simulink model "siasun_config_casadi_VS_lsj_sim_16a"  (R2020a)
settings: Solver=FixedStepAuto  StartTime=0.0  StopTime=20  FixedStep=0.001  RelTol=1e-3  EnableMultiTasking=on
values from neighbouring files (symbols this model uses):
  a1 = 0.040    (= 0.04)    [set_mode_parameter_siasun.m]
  a2 = 0.275    [set_mode_parameter_siasun.m]
  a3 = 0.025    [set_mode_parameter_siasun.m]
  d1 = 0.342    [set_mode_parameter_siasun.m]
  d4 = 0.280    (= 0.28)    [set_mode_parameter_siasun.m]
  fc1 = 0    [set_mode_parameter_siasun.m]
  fc2 = 0    [set_mode_parameter_siasun.m]
  fc3 = 0    [set_mode_parameter_siasun.m]
  fc4 = 0    [set_mode_parameter_siasun.m]
  fc5 = 0    [set_mode_parameter_siasun.m]
  fc6 = 0    [set_mode_parameter_siasun.m]
  fv1 = 0    [set_mode_parameter_siasun.m]
  fv2 = 0    [set_mode_parameter_siasun.m]
  fv3 = 0    [set_mode_parameter_siasun.m]
  fv4 = 0    [set_mode_parameter_siasun.m]
  fv5 = 0    [set_mode_parameter_siasun.m]
  fv6 = 0    [set_mode_parameter_siasun.m]
  Ia1 = 0    [set_mode_parameter_siasun.m]
  Ia2 = 0    [set_mode_parameter_siasun.m]
  Ia3 = 0    [set_mode_parameter_siasun.m]
  Ia4 = 0    [set_mode_parameter_siasun.m]
  Ia5 = 0    [set_mode_parameter_siasun.m]
  Ia6 = 0    [set_mode_parameter_siasun.m]
  Ic111 = 0    [set_mode_parameter_siasun.m]
  Ic112 = 0    [set_mode_parameter_siasun.m]
  Ic113 = 0    [set_mode_parameter_siasun.m]
  Ic122 = 0    [set_mode_parameter_siasun.m]
  Ic123 = 0    [set_mode_parameter_siasun.m]
  Ic133 = 1.3676    [set_mode_parameter_siasun.m]
  Ic211 = 8.8194    [set_mode_parameter_siasun.m]
  Ic212 = 0    [set_mode_parameter_siasun.m]
  Ic213 = 0    [set_mode_parameter_siasun.m]
  Ic222 = 6.0549    [set_mode_parameter_siasun.m]
  Ic223 = 0    [set_mode_parameter_siasun.m]
  Ic233 = 0.9569    [set_mode_parameter_siasun.m]
  Ic311 = 0.0332    [set_mode_parameter_siasun.m]
  Ic312 = 0    [set_mode_parameter_siasun.m]
  Ic313 = 0    [set_mode_parameter_siasun.m]
  Ic322 = 1.8442    [set_mode_parameter_siasun.m]
  Ic323 = 0    [set_mode_parameter_siasun.m]
  Ic333 = 1.0560    (= 1.056)    [set_mode_parameter_siasun.m]
  Ic411 = 0.1448    [set_mode_parameter_siasun.m]
  Ic412 = 0    [set_mode_parameter_siasun.m]
  Ic413 = 0    [set_mode_parameter_siasun.m]
  Ic422 = 0.0015    [set_mode_parameter_siasun.m]
  Ic423 = 0    [set_mode_parameter_siasun.m]
  Ic433 = 0.0822    [set_mode_parameter_siasun.m]
  Ic511 = 0    [set_mode_parameter_siasun.m]
  Ic512 = 0    [set_mode_parameter_siasun.m]
  Ic513 = 0    [set_mode_parameter_siasun.m]
  Ic522 = 0.0121    [set_mode_parameter_siasun.m]
  Ic523 = 0    [set_mode_parameter_siasun.m]
  Ic533 = 0.0299    [set_mode_parameter_siasun.m]
  Ic611 = 0.0134    [set_mode_parameter_siasun.m]
  Ic612 = 0    [set_mode_parameter_siasun.m]
  Ic613 = 0    [set_mode_parameter_siasun.m]
  Ic622 = 0    [set_mode_parameter_siasun.m]
  Ic623 = 0    [set_mode_parameter_siasun.m]
  Ic633 = 0.0051    [set_mode_parameter_siasun.m]
  m1 = 0.167    [set_mode_parameter_siasun.m]
  m2 = 1    [set_mode_parameter_siasun.m]
  m3 = 0.5    [set_mode_parameter_siasun.m]
  m4 = 0.333    [set_mode_parameter_siasun.m]
  m5 = 0.25    [set_mode_parameter_siasun.m]
  m6 = 0.2    [set_mode_parameter_siasun.m]
  mc11 = 0    [set_mode_parameter_siasun.m]
  mc12 = 0    [set_mode_parameter_siasun.m]
  mc13 = 0.2    [set_mode_parameter_siasun.m]
  mc21 = 0.1291    [set_mode_parameter_siasun.m]
  mc22 = 0    [set_mode_parameter_siasun.m]
  mc23 = 3.3117    [set_mode_parameter_siasun.m]
  mc31 = 1.6484    [set_mode_parameter_siasun.m]
  mc32 = 0    [set_mode_parameter_siasun.m]
  mc33 = 0.8748    [set_mode_parameter_siasun.m]
  mc41 = 0.3200    (= 0.32)    [set_mode_parameter_siasun.m]
  mc42 = 0.2324    [set_mode_parameter_siasun.m]
  mc43 = 0.7083    [set_mode_parameter_siasun.m]
  mc51 = 0.4574    [set_mode_parameter_siasun.m]
  mc52 = 0    [set_mode_parameter_siasun.m]
  mc53 = 0.6427    [set_mode_parameter_siasun.m]
  mc61 = 0.3200    (= 0.32)    [set_mode_parameter_siasun.m]
  mc62 = -0.0513    [set_mode_parameter_siasun.m]
  mc63 = 0.6417    [set_mode_parameter_siasun.m]
undefined symbols (not defined in the file or in its folder): X, Y, Z
libraries: sm_lib x224, nesl_utility x124, simulink x8
(part 6 of 11)

== system siasun_config_casadi_VS_lsj_sim_16a/xb4_rel/Robot/Robot/robot/link6 ==
  Inertia : sm_lib/Body Elements/Inertia  InertiaType=Custom  Mass=m6  MassUnits=kg  CenterOfMass=[mc61 mc62 mc63]  CenterOfMassUnits=m  MomentsOfInertia=[Ic611 Ic622 Ic633 ]  MomentsOfInertiaUnits=kg*m^2  ProductsOfInertia=[Ic623 Ic613 Ic612]  ProductsOfInertiaUnits=kg*m^2  GraphicType=Marker  MarkerShape=Inertia  MarkerSize=20  GraphicVisPropType=SimpleVisualProperties  GraphicDiffuseColor=[0.5 0.5 0.5]  GraphicSpecularColor=[0.5 0.5 0.5 1.0]  GraphicAmbientColor=[0.15 0.15 0.15 1.0]  GraphicEmissiveColor=[0.0 0.0 0.0 1.0]  GraphicShininess=75  GraphicOpacity=1.0
  Reference Frame : sm_lib/Frames and Transforms/Reference Frame
  base : sm_lib/Body Elements/File Solid  ExtGeomFileName=XB4_Model\XB4-6.STL  UnitType=Custom  ExtGeomFileUnits=mm  StepReaderType=HEX  ExportConvexHullGeometry=off  InertiaType=Custom  Mass=0  MassUnits=kg  CenterOfMass=[0 0 0]  CenterOfMassUnits=m  MomentsOfInertia=[0 0 0]  MomentsOfInertiaUnits=kg*m^2  ProductsOfInertia=[0 0 0]  ProductsOfInertiaUnits=kg*m^2  BasedOnType=Density  Density=1000  DensityUnits=kg/(m^3)  DoExposeReferenceFrame=on  SerializedFrames=<Frames/>  GraphicType=FromGeometry  MarkerShape=Sphere  MarkerSize=10  GraphicVisPropType=SimpleVisualProperties  GraphicDiffuseColor=[0.5 0.5 0.5]  GraphicSpecularColor=[0.5 0.5 0.5 1.0]  GraphicAmbientColor=[0.15 0.15 0.15 1.0]  GraphicEmissiveColor=[0.0 0.0 0.0 1.0]  GraphicShininess=75  GraphicOpacity=1.0
  joint1_OriginTransform1 : sm_lib/Frames and Transforms/Rigid Transform  TranslationMethod=Cartesian  TranslationStandardOffset=0  TranslationLengthUnit=m  TranslationStandardAxis=+Z  TranslationCartesianOffset=[0 0 d1]  TranslationROffset=0  TranslationROffsetUnits=m  TranslationZOffset=0  TranslationZOffsetUnits=m  TranslationThetaOffset=0  TranslationThetaOffsetUnits=deg  RotationMethod=RotationSequence  RotationAngleUnits=deg  RotationStandardAxis=+Z  RotationAngle=0.0  RotationArbitraryAxis=[0 0 1]  FollAlignAxisA=+X  BaseAlignAxisA=+Y  FollAlignAxisB=+Y  BaseAlignAxisB=+Z  RotationSequenceAxes=BaseAxes  RotationSequence=XYZ  RotationSequenceAngles=[0 0 0]  RotationSequenceAnglesUnits=rad  RotationMatrix=[1 0 0; 0 1 0; 0 0 1]
  joint2_OriginTransform1 : sm_lib/Frames and Transforms/Rigid Transform  TranslationMethod=Cartesian  TranslationStandardOffset=0  TranslationLengthUnit=m  TranslationStandardAxis=+Z  TranslationCartesianOffset=[a1 0 0]  TranslationROffset=0  TranslationROffsetUnits=m  TranslationZOffset=0  TranslationZOffsetUnits=m  TranslationThetaOffset=0  TranslationThetaOffsetUnits=deg  RotationMethod=RotationSequence  RotationAngleUnits=deg  RotationStandardAxis=+Z  RotationAngle=0.0  RotationArbitraryAxis=[0 0 1]  FollAlignAxisA=+X  BaseAlignAxisA=+Y  FollAlignAxisB=+Y  BaseAlignAxisB=+Z  RotationSequenceAxes=FollowerAxes  RotationSequence=XYZ  RotationSequenceAngles=[-pi/2 0 -pi/2]  RotationSequenceAnglesUnits=rad  RotationMatrix=[1 0 0; 0 1 0; 0 0 1]
  joint3_OriginTransform1 : sm_lib/Frames and Transforms/Rigid Transform  TranslationMethod=Cartesian  TranslationStandardOffset=0  TranslationLengthUnit=m  TranslationStandardAxis=+Z  TranslationCartesianOffset=[a2 0 0]  TranslationROffset=0  TranslationROffsetUnits=m  TranslationZOffset=0  TranslationZOffsetUnits=m  TranslationThetaOffset=0  TranslationThetaOffsetUnits=deg  RotationMethod=RotationSequence  RotationAngleUnits=deg  RotationStandardAxis=+Z  RotationAngle=0.0  RotationArbitraryAxis=[0 0 1]  FollAlignAxisA=+X  BaseAlignAxisA=+Y  FollAlignAxisB=+Y  BaseAlignAxisB=+Z  RotationSequenceAxes=FollowerAxes  RotationSequence=XYZ  RotationSequenceAngles=[0 0 0]  RotationSequenceAnglesUnits=rad  RotationMatrix=[1 0 0; 0 1 0; 0 0 1]
  joint4_AxisInvTransform : sm_lib/Frames and Transforms/Rigid Transform  TranslationMethod=Cartesian  TranslationStandardOffset=0  TranslationLengthUnit=m  TranslationStandardAxis=+Z  TranslationCartesianOffset=[0 0 0]  TranslationROffset=0  TranslationROffsetUnits=m  TranslationZOffset=0  TranslationZOffsetUnits=m  TranslationThetaOffset=0  TranslationThetaOffsetUnits=deg  RotationMethod=RotationSequence  RotationAngleUnits=rad  RotationStandardAxis=+Z  RotationAngle=1.570796  RotationArbitraryAxis=[0 1 0]  FollAlignAxisA=+X  BaseAlignAxisA=+Y  FollAlignAxisB=+Y  BaseAlignAxisB=+Z  RotationSequenceAxes=FollowerAxes  RotationSequence=XYZ  RotationSequenceAngles=[pi/2 0 0]  RotationSequenceAnglesUnits=rad  RotationMatrix=[1 0 0; 0 1 0; 0 0 1]
  joint4_OriginTransform1 : sm_lib/Frames and Transforms/Rigid Transform  TranslationMethod=Cartesian  TranslationStandardOffset=0  TranslationLengthUnit=m  TranslationStandardAxis=+Z  TranslationCartesianOffset=[a3 d4 0]  TranslationROffset=0  TranslationROffsetUnits=m  TranslationZOffset=0  TranslationZOffsetUnits=m  TranslationThetaOffset=0  TranslationThetaOffsetUnits=deg  RotationMethod=RotationSequence  RotationAngleUnits=deg  RotationStandardAxis=+Z  RotationAngle=0.0  RotationArbitraryAxis=[0 0 1]  FollAlignAxisA=+X  BaseAlignAxisA=+Y  FollAlignAxisB=+Y  BaseAlignAxisB=+Z  RotationSequenceAxes=FollowerAxes  RotationSequence=XYZ  RotationSequenceAngles=[-pi/2 0 0]  RotationSequenceAnglesUnits=rad  RotationMatrix=[1 0 0; 0 1 0; 0 0 1]
  joint6_OriginTransform1 : sm_lib/Frames and Transforms/Rigid Transform  TranslationMethod=Cartesian  TranslationStandardOffset=0  TranslationLengthUnit=m  TranslationStandardAxis=+Z  TranslationCartesianOffset=[0 0 0]  TranslationROffset=0  TranslationROffsetUnits=m  TranslationZOffset=0  TranslationZOffsetUnits=m  TranslationThetaOffset=0  TranslationThetaOffsetUnits=deg  RotationMethod=RotationSequence  RotationAngleUnits=deg  RotationStandardAxis=+Z  RotationAngle=0.0  RotationArbitraryAxis=[0 0 1]  FollAlignAxisA=+X  BaseAlignAxisA=+Y  FollAlignAxisB=+Y  BaseAlignAxisB=+Z  RotationSequenceAxes=FollowerAxes  RotationSequence=XYZ  RotationSequenceAngles=[-pi/2 0 0]  RotationSequenceAnglesUnits=rad  RotationMatrix=[1 0 0; 0 1 0; 0 0 1]
  F : PMIOPort  Side=Left
  connections:
  Reference Frame/RConn1 -- joint6_OriginTransform1/RConn1 -- Inertia/RConn1 -- F/RConn1
  joint6_OriginTransform1/LConn1 -- joint4_AxisInvTransform/RConn1
  joint1_OriginTransform1/LConn1 -- base/RConn1
  joint3_OriginTransform1/LConn1 -- joint2_OriginTransform1/RConn1
  joint4_OriginTransform1/RConn1 -- joint4_AxisInvTransform/LConn1
  joint4_OriginTransform1/LConn1 -- joint3_OriginTransform1/RConn1
  joint2_OriginTransform1/LConn1 -- joint1_OriginTransform1/RConn1

== matlab function siasun_config_casadi_VS_lsj_sim_16a/xb4_obs/Robot/Robot/robot/friction ==
  data: u input; y output; fv input; fc input
function y = fcn(u,fv,fc)
%#codegen


% fv1=100; fc1=80; fv2=150; fc2=100; fv3=100; fc3=50; fv4=80; fc4=80; fv5=50; fc5=30; fv6=30; fc6=10;
fv1=fv(1); fc1=fc(1); fv2=fv(2); fc2=fc(2); fv3=fv(3); fc3=fc(3); fv4=fv(4); fc4=fc(4); fv5=fv(5); fc5=fc(5); fv6=fv(6); fc6=fc(6);
y=[0;0;0;0;0;0];
y(1)=(fv1*u(1)+fc1*sign(u(1)));
y(2)=(fv2*u(2)+fc2*sign(u(2)));
y(3)=(fv3*u(3)+fc3*sign(u(3)));
y(4)=(fv4*u(4)+fc4*sign(u(4)));
y(5)=(fv5*u(5)+fc5*sign(u(5)));
y(6)=(fv6*u(6)+fc6*sign(u(6)));

end

== matlab function siasun_config_casadi_VS_lsj_sim_16a/DH-IK4 ==
  data: angle1 input; t input; Radian output; angle2 input
function Radian  = read(angle1,t,angle2)
if t <= 5
    Radian = angle2;
else
    Radian = angle1;
end
end

== matlab function siasun_config_casadi_VS_lsj_sim_16a/三阶曲线规划1/一关节/3_planning1 ==
  data: state output; plan3_A output; g_vs parameter; g_ve parameter; S input; tf input; tf output
function [state, plan3_A,tf] =planning3( g_vs, g_ve,S,tf)
% 三次多项式算法主程序
% vs初始速度m/min,ve末速度m/min,S总位移m,
% 基础插补规划函数
% 三次多项式速度规划
    a0 = 0 ;
    a1 = g_vs ;
    a2 = 3*S/tf^2 - 2* g_vs/tf - g_ve/tf;
    a3 = -2*S/tf^3 - (g_vs+g_ve)/tf^2;
    state = 1;
    plan3_A = [a0 a1 a2 a3];
    tf =tf ;

end

== matlab function siasun_config_casadi_VS_lsj_sim_16a/三阶曲线规划1/一关节/Interpolation3 ==
  data: state output; Enable input; Y output; plan3_A input; tf input; t input
function [state, Y]  = Interpolate3(Enable,plan3_A,tf,t)
%% input
a0 = plan3_A(1);
a1 = plan3_A(2);
a2 = plan3_A(3);
a3 = plan3_A(4);
Y = 0;
%% output
if Enable == 1
    if t <=tf
    Y = a0 + a1*t + a2*t^2 + a3*t^3; 
    state =1;
    else
    Y = a0 + a1*tf + a2*tf^2 + a3*tf^3;
    state = 1;
    end
else 
    Y = 0;
    state = 0;
end
end

== matlab function siasun_config_casadi_VS_lsj_sim_16a/三阶曲线规划1/三关节/3_planning1 ==
  data: state output; plan3_A output; g_vs parameter; g_ve parameter; S input; tf input; tf output
function [state, plan3_A,tf] =planning3( g_vs, g_ve,S,tf)
% 三次多项式算法主程序
% vs初始速度m/min,ve末速度m/min,S总位移m,
% 基础插补规划函数
% 三次多项式速度规划
    a0 = 0 ;
    a1 = g_vs ;
    a2 = 3*S/tf^2 - 2* g_vs/tf - g_ve/tf;
    a3 = -2*S/tf^3 - (g_vs+g_ve)/tf^2;
    state = 1;
    plan3_A = [a0 a1 a2 a3];
    tf =tf ;

end

== matlab function siasun_config_casadi_VS_lsj_sim_16a/三阶曲线规划1/二关节/3_planning1 ==
  data: state output; plan3_A output; g_vs parameter; g_ve parameter; S input; tf input; tf output
function [state, plan3_A,tf] =planning3( g_vs, g_ve,S,tf)
% 三次多项式算法主程序
% vs初始速度m/min,ve末速度m/min,S总位移m,
% 基础插补规划函数
% 三次多项式速度规划
    a0 = 0 ;
    a1 = g_vs ;
    a2 = 3*S/tf^2 - 2* g_vs/tf - g_ve/tf;
    a3 = -2*S/tf^3 - (g_vs+g_ve)/tf^2;
    state = 1;
    plan3_A = [a0 a1 a2 a3];
    tf =tf ;

end

== matlab function siasun_config_casadi_VS_lsj_sim_16a/三阶曲线规划1/二关节/Interpolation3 ==
  data: state output; Enable input; Y output; plan3_A input; tf input; t input
function [state, Y]  = Interpolate3(Enable,plan3_A,tf,t)
%% input
a0 = plan3_A(1);
a1 = plan3_A(2);
a2 = plan3_A(3);
a3 = plan3_A(4);
Y = 0;
%% output
if Enable == 1
    if t <=tf
    Y = a0 + a1*t + a2*t^2 + a3*t^3; 
    state =1;
    else
    Y = a0 + a1*tf + a2*tf^2 + a3*tf^3;
    state = 1;
    end
else 
    Y = 0;
    state = 0;
end
end

== matlab function siasun_config_casadi_VS_lsj_sim_16a/三阶曲线规划1/五关节/3_planning1 ==
  data: state output; plan3_A output; g_vs parameter; g_ve parameter; S input; tf input; tf output
function [state, plan3_A,tf] =planning3( g_vs, g_ve,S,tf)
% 三次多项式算法主程序
% vs初始速度m/min,ve末速度m/min,S总位移m,
% 基础插补规划函数
% 三次多项式速度规划
    a0 = 0 ;
    a1 = g_vs ;
    a2 = 3*S/tf^2 - 2* g_vs/tf - g_ve/tf;
    a3 = -2*S/tf^3 - (g_vs+g_ve)/tf^2;
    state = 1;
    plan3_A = [a0 a1 a2 a3];
    tf =tf ;

end

== matlab function siasun_config_casadi_VS_lsj_sim_16a/三阶曲线规划1/三关节/Interpolation3 ==
  data: state output; Enable input; Y output; plan3_A input; tf input; t input
function [state, Y]  = Interpolate3(Enable,plan3_A,tf,t)
%% input
a0 = plan3_A(1);
a1 = plan3_A(2);
a2 = plan3_A(3);
a3 = plan3_A(4);
Y = 0;
%% output
if Enable == 1
    if t <=tf
    Y = a0 + a1*t + a2*t^2 + a3*t^3; 
    state =1;
    else
    Y = a0 + a1*tf + a2*tf^2 + a3*tf^3;
    state = 1;
    end
else 
    Y = 0;
    state = 0;
end
end

== matlab function siasun_config_casadi_VS_lsj_sim_16a/三阶曲线规划1/五关节/Interpolation3 ==
  data: state output; Enable input; Y output; plan3_A input; tf input; t input
function [state, Y]  = Interpolate3(Enable,plan3_A,tf,t)
%% input
a0 = plan3_A(1);
a1 = plan3_A(2);
a2 = plan3_A(3);
a3 = plan3_A(4);
Y = 0;
%% output
if Enable == 1
    if t <=tf
    Y = a0 + a1*t + a2*t^2 + a3*t^3; 
    state =1;
    else
    Y = a0 + a1*tf + a2*tf^2 + a3*tf^3;
    state = 1;
    end
else 
    Y = 0;
    state = 0;
end
end

== matlab function siasun_config_casadi_VS_lsj_sim_16a/三阶曲线规划1/六关节/3_planning1 ==
  data: state output; plan3_A output; g_vs parameter; g_ve parameter; S input; tf input; tf output
function [state, plan3_A,tf] =planning3( g_vs, g_ve,S,tf)
% 三次多项式算法主程序
% vs初始速度m/min,ve末速度m/min,S总位移m,
% 基础插补规划函数
% 三次多项式速度规划
    a0 = 0 ;
    a1 = g_vs ;
    a2 = 3*S/tf^2 - 2* g_vs/tf - g_ve/tf;
    a3 = -2*S/tf^3 - (g_vs+g_ve)/tf^2;
    state = 1;
    plan3_A = [a0 a1 a2 a3];
    tf =tf ;

end

== matlab function siasun_config_casadi_VS_lsj_sim_16a/三阶曲线规划1/六关节/Interpolation3 ==
  data: state output; Enable input; Y output; plan3_A input; tf input; t input
function [state, Y]  = Interpolate3(Enable,plan3_A,tf,t)
%% input
a0 = plan3_A(1);
a1 = plan3_A(2);
a2 = plan3_A(3);
a3 = plan3_A(4);
Y = 0;
%% output
if Enable == 1
    if t <=tf
    Y = a0 + a1*t + a2*t^2 + a3*t^3; 
    state =1;
    else
    Y = a0 + a1*tf + a2*tf^2 + a3*tf^3;
    state = 1;
    end
else 
    Y = 0;
    state = 0;
end
end

== matlab function siasun_config_casadi_VS_lsj_sim_16a/三阶曲线规划1/四关节/3_planning1 ==
  data: state output; plan3_A output; g_vs parameter; g_ve parameter; S input; tf input; tf output
function [state, plan3_A,tf] =planning3( g_vs, g_ve,S,tf)
% 三次多项式算法主程序
% vs初始速度m/min,ve末速度m/min,S总位移m,
% 基础插补规划函数
% 三次多项式速度规划
    a0 = 0 ;
    a1 = g_vs ;
    a2 = 3*S/tf^2 - 2* g_vs/tf - g_ve/tf;
    a3 = -2*S/tf^3 - (g_vs+g_ve)/tf^2;
    state = 1;
    plan3_A = [a0 a1 a2 a3];
    tf =tf ;

end

== matlab function siasun_config_casadi_VS_lsj_sim_16a/siasun_rel/Robot/Robot/robot/Jm ==
  data: u input; y output; Jm input
function y = fcn(u,Jm)
%#codegen

% Jm=[200; 250; 150; 100; 50; 20];%关节惯性
y = Jm.*u;
end

== matlab function siasun_config_casadi_VS_lsj_sim_16a/三阶曲线规划1/四关节/Interpolation3 ==
  data: state output; Enable input; Y output; plan3_A input; tf input; t input
function [state, Y]  = Interpolate3(Enable,plan3_A,tf,t)
%% input
a0 = plan3_A(1);
a1 = plan3_A(2);
a2 = plan3_A(3);
a3 = plan3_A(4);
Y = 0;
%% output
if Enable == 1
    if t <=tf
    Y = a0 + a1*t + a2*t^2 + a3*t^3; 
    state =1;
    else
    Y = a0 + a1*tf + a2*tf^2 + a3*tf^3;
    state = 1;
    end
else 
    Y = 0;
    state = 0;
end
end

== matlab function siasun_config_casadi_VS_lsj_sim_16a/xb4_rel/Robot/Robot/robot/Jm ==
  data: u input; y output; Jm input
function y = fcn(u,Jm)
%#codegen

% Jm=[200; 250; 150; 100; 50; 20];%关节惯性
y = Jm.*u;
end

== matlab function siasun_config_casadi_VS_lsj_sim_16a/xb4_rel/Robot/Robot/robot/friction ==
  data: u input; y output; fv input; fc input
function y = fcn(u,fv,fc)
%#codegen


% fv1=100; fc1=80; fv2=150; fc2=100; fv3=100; fc3=50; fv4=80; fc4=80; fv5=50; fc5=30; fv6=30; fc6=10;
fv1=fv(1); fc1=fc(1); fv2=fv(2); fc2=fc(2); fv3=fv(3); fc3=fc(3); fv4=fv(4); fc4=fc(4); fv5=fv(5); fc5=fc(5); fv6=fv(6); fc6=fc(6);
y=[0;0;0;0;0;0];
y(1)=(fv1*u(1)+fc1*sign(u(1)));
y(2)=(fv2*u(2)+fc2*sign(u(2)));
y(3)=(fv3*u(3)+fc3*sign(u(3)));
y(4)=(fv4*u(4)+fc4*sign(u(4)));
y(5)=(fv5*u(5)+fc5*sign(u(5)));
y(6)=(fv6*u(6)+fc6*sign(u(6)));

end
